simulink model "SEND_TEST"  (R2021b)
settings: Solver=VariableStepAuto  StartTime=0.0  StopTime=inf  RelTol=1e-3
libraries: instrumentlib x4
settings Model: Creator=ccortes9  LastModifiedBy=ccortes9

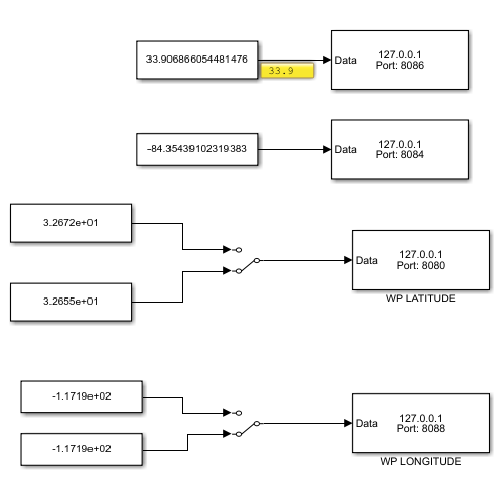
[thumbnail: Simulink's stored preview of the top-level diagram]
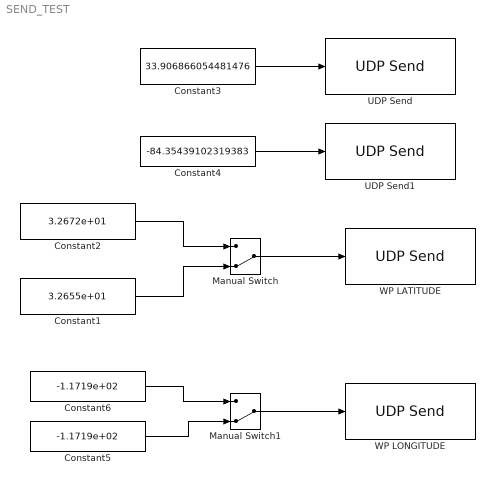
== system SEND_TEST ==
  Constant1 : Constant  Value=3.2655e+01  SampleTime=0.01
  Constant2 : Constant  Value=3.2672e+01  SampleTime=0.01
  Constant3 : Constant  Value=33.906866054481476  SampleTime=0.01
  Constant4 : Constant  Value=-84.35439102319383  SampleTime=0.01
  Constant5 : Constant  Value=-1.1719e+02  SampleTime=0.01
  Constant6 : Constant  Value=-1.1719e+02  SampleTime=0.01
  Manual Switch : ManualSwitch  CurrentSetting=0
  Manual Switch1 : ManualSwitch  CurrentSetting=0
  UDP Send : instrumentlib/UDP Send  Host=127.0.0.1  Port=8086  LocalPort=8081  EnablePortSharing=off  ByteOrder=BigEndian  OutputDatagramPacketSize=512  EnableBlockingMode=on  LocalAddress=127.0.0.1
  UDP Send1 : instrumentlib/UDP Send  Host=127.0.0.1  Port=8084  LocalPort=8083  EnablePortSharing=off  ByteOrder=BigEndian  OutputDatagramPacketSize=512  EnableBlockingMode=on  LocalAddress=127.0.0.1
  WP LATITUDE : instrumentlib/UDP Send  Host=127.0.0.1  Port=8080  LocalPort=8087  EnablePortSharing=off  ByteOrder=BigEndian  OutputDatagramPacketSize=512  EnableBlockingMode=on  LocalAddress=127.0.0.1
  WP LONGITUDE : instrumentlib/UDP Send  Host=127.0.0.1  Port=8088  LocalPort=8089  EnablePortSharing=off  ByteOrder=BigEndian  OutputDatagramPacketSize=512  EnableBlockingMode=on  LocalAddress=127.0.0.1
  wires:
  Constant4/1 -> UDP Send1/1
  Constant3/1 -> UDP Send/1
  Constant5/1 -> Manual Switch1/2
  Constant1/1 -> Manual Switch/2
  Manual Switch1/1 -> WP LONGITUDE/1
  Manual Switch/1 -> WP LATITUDE/1
  Constant2/1 -> Manual Switch/1
  Constant6/1 -> Manual Switch1/1
